simulink library "car_library"  (R2019b)
settings: Solver=VariableStepAuto  StartTime=0.0  StopTime=10.0  RelTol=1e-3
undefined symbols (not defined in the file): car, car_init
libraries: simulink x2, $bdroot x2
settings Model: Creator=ciba  LastModifiedBy=LongLongMagnumDong
settings DataIOCC: ReturnWorkspaceOutputs=off
settings DebuggingCC: ArithmeticOperatorsInVariantConditions=warning
settings SFSimCC: SimUseLocalCustomCode=off  CustomCodeUndefinedFunction=UseInterfaceOnly
settings RTWCC: RTWUseLocalCustomCode=off
settings CodeAppCC: StateflowObjectComments=on

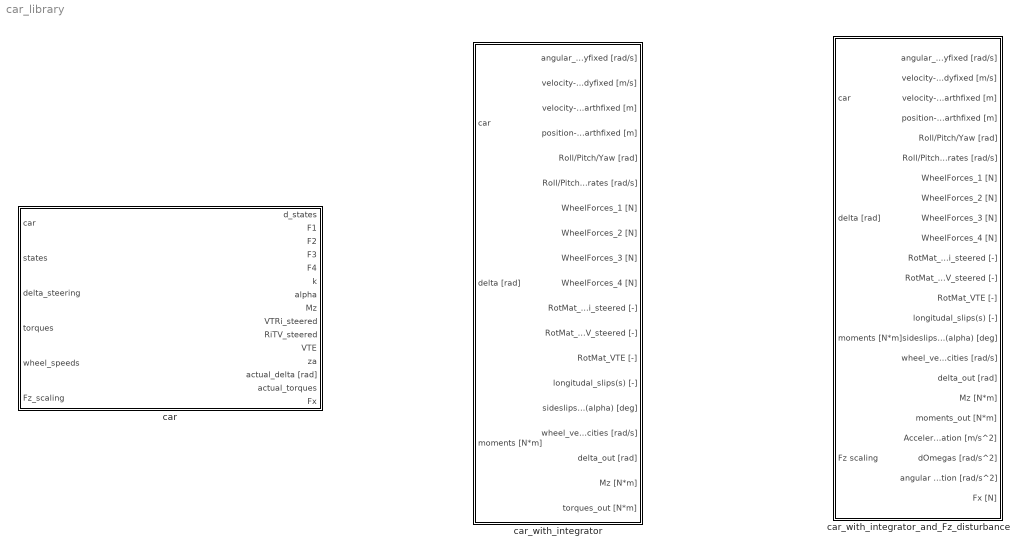
== system car_library ==
  car : Subsystem
  car_with_integrator : Subsystem
  car_with_integrator_and_Fz_disturbance : Subsystem

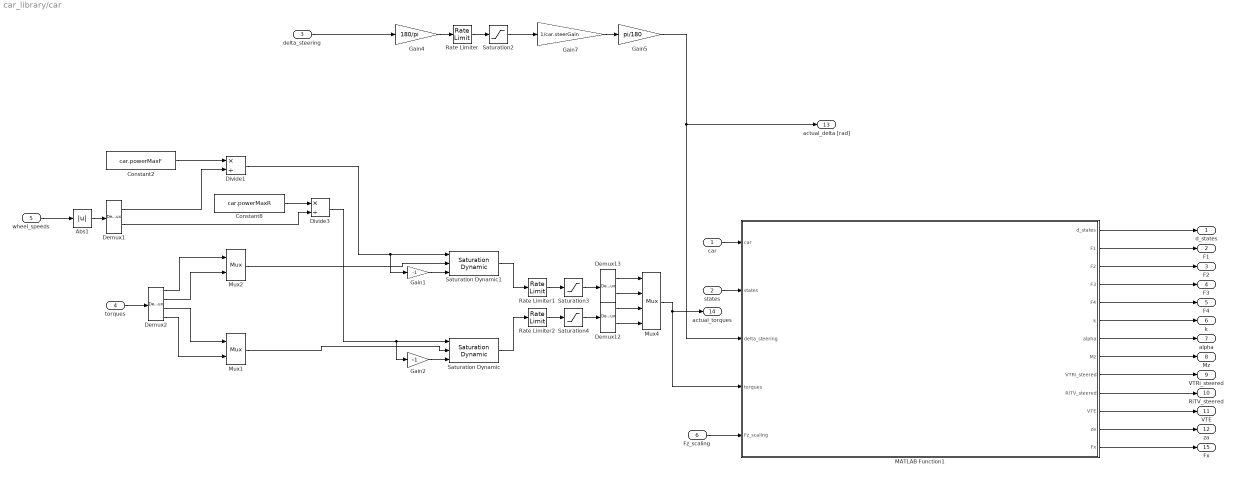
== system car_library/car ==
  car : Inport
  states : Inport  Port=2
  delta_steering : Inport  Port=3  PortDimensions=4
  torques : Inport  Port=4
  wheel_speeds : Inport  Port=5
  Fz_scaling : Inport  Port=6
  Abs1 : Abs
  Constant2 : Constant  Value=car.powerMaxF
  Constant8 : Constant  Value=car.powerMaxR
  Demux1 : Demux  Outputs=2
  Demux12 : Demux  Outputs=2
  Demux13 : Demux  Outputs=2
  Demux2 : Demux
  Divide1 : Product  Inputs=*/
  Divide3 : Product  Inputs=*/
  Gain1 : Gain  Gain=-1
  Gain2 : Gain  Gain=-1
  Gain4 : Gain  Gain=180/pi
  Gain5 : Gain  Gain=pi/180
  Gain7 : Gain  Gain=1/car.steerGain
  MATLAB Function1 : MATLAB Function  TreatAsAtomicUnit=on
  Mux1 : Mux  Inputs=2
  Mux2 : Mux  Inputs=2
  Mux4 : Mux
  Rate Limiter : RateLimiter  RisingSlewLimit=car.steerRate  FallingSlewLimit=-car.steerRate  SampleTimeMode=inherited
  Rate Limiter1 : RateLimiter  RisingSlewLimit=car.torqueRate  FallingSlewLimit=-car.torqueRate  SampleTimeMode=inherited
  Rate Limiter2 : RateLimiter  RisingSlewLimit=car.torqueRate  FallingSlewLimit=-car.torqueRate  SampleTimeMode=inherited
  Saturation Dynamic : simulink/Discontinuities/Saturation Dynamic  OutMin=[]  OutMax=[]  OutDataTypeStr=Inherit: Same as second input  OutDataType=fixdt(1, 16)  OutScaling=2^-10  DoSatur=off
  Saturation Dynamic1 : simulink/Discontinuities/Saturation Dynamic  OutMin=[]  OutMax=[]  OutDataTypeStr=Inherit: Same as second input  OutDataType=fixdt(1, 16)  OutScaling=2^-10  DoSatur=off
  Saturation2 : Saturate  UpperLimit=car.steerMaxDeg  LowerLimit=-car.steerMaxDeg
  Saturation3 : Saturate  UpperLimit=car.torqueMaxF  LowerLimit=-car.torqueMaxF
  Saturation4 : Saturate  UpperLimit=car.torqueMaxR  LowerLimit=-car.torqueMaxR
  d_states : Outport  VectorParamsAs1DForOutWhenUnconnected=off
  F1 : Outport  Port=2  VectorParamsAs1DForOutWhenUnconnected=off
  F2 : Outport  Port=3  VectorParamsAs1DForOutWhenUnconnected=off
  F3 : Outport  Port=4  VectorParamsAs1DForOutWhenUnconnected=off
  F4 : Outport  Port=5  VectorParamsAs1DForOutWhenUnconnected=off
  k : Outport  Port=6  VectorParamsAs1DForOutWhenUnconnected=off
  alpha : Outport  Port=7  VectorParamsAs1DForOutWhenUnconnected=off
  Mz : Outport  Port=8  VectorParamsAs1DForOutWhenUnconnected=off
  VTRi_steered : Outport  Port=9  VectorParamsAs1DForOutWhenUnconnected=off
  RiTV_steered : Outport  Port=10  VectorParamsAs1DForOutWhenUnconnected=off
  VTE : Outport  Port=11  VectorParamsAs1DForOutWhenUnconnected=off
  za : Outport  Port=12  VectorParamsAs1DForOutWhenUnconnected=off
  actual_delta [rad] : Outport  Port=13  VectorParamsAs1DForOutWhenUnconnected=off
  actual_torques : Outport  Port=14  VectorParamsAs1DForOutWhenUnconnected=off
  Fx : Outport  Port=15  VectorParamsAs1DForOutWhenUnconnected=off
  wires:
  Rate Limiter2/1 -> Saturation4/1
  Demux12/1 -> Mux4/3
  Saturation3/1 -> Demux13/1
  Demux1/2 -> Divide3/2
  Saturation4/1 -> Demux12/1
  Mux1/1 -> Saturation Dynamic/2
  Demux12/2 -> Mux4/4
  Demux2/1 -> Mux2/1
  Demux13/1 -> Mux4/1
  Saturation Dynamic/1 -> Rate Limiter2/1
  Rate Limiter1/1 -> Saturation3/1
  Demux13/2 -> Mux4/2
  Constant8/1 -> Divide3/1
  Abs1/1 -> Demux1/1
  Mux4/1 -> MATLAB Function1/4(torques), actual_torques/1
  car/1 -> MATLAB Function1/1(car)
  states/1 -> MATLAB Function1/2(states)
  MATLAB Function1/2(F1) -> F1/1
  MATLAB Function1/6(k) -> k/1
  MATLAB Function1/12(za) -> za/1
  MATLAB Function1/10(RiTV_steered) -> RiTV_steered/1
  MATLAB Function1/11(VTE) -> VTE/1
  MATLAB Function1/4(F3) -> F3/1
  torques/1 -> Demux2/1
  MATLAB Function1/1(d_states) -> d_states/1
  MATLAB Function1/3(F2) -> F2/1
  MATLAB Function1/9(VTRi_steered) -> VTRi_steered/1
  MATLAB Function1/8(Mz) -> Mz/1
  MATLAB Function1/5(F4) -> F4/1
  MATLAB Function1/7(alpha) -> alpha/1
  Demux2/4 -> Mux1/2
  Saturation Dynamic1/1 -> Rate Limiter1/1
  Mux2/1 -> Saturation Dynamic1/2
  Demux2/2 -> Mux2/2
  Constant2/1 -> Divide1/1
  Divide1/1 -> Gain1/1, Saturation Dynamic1/1
  wheel_speeds/1 -> Abs1/1
  Demux2/3 -> Mux1/1
  Gain4/1 -> Rate Limiter/1
  delta_steering/1 -> Gain4/1
  Saturation2/1 -> Gain7/1
  Rate Limiter/1 -> Saturation2/1
  Gain7/1 -> Gain5/1
  Gain1/1 -> Saturation Dynamic1/3
  Divide3/1 -> Gain2/1, Saturation Dynamic/1
  Gain2/1 -> Saturation Dynamic/3
  Demux1/1 -> Divide1/2
  Gain5/1 -> actual_delta [rad]/1, MATLAB Function1/3(delta_steering)
  Fz_scaling/1 -> MATLAB Function1/5(Fz_scaling)
  MATLAB Function1/13(Fx) -> Fx/1

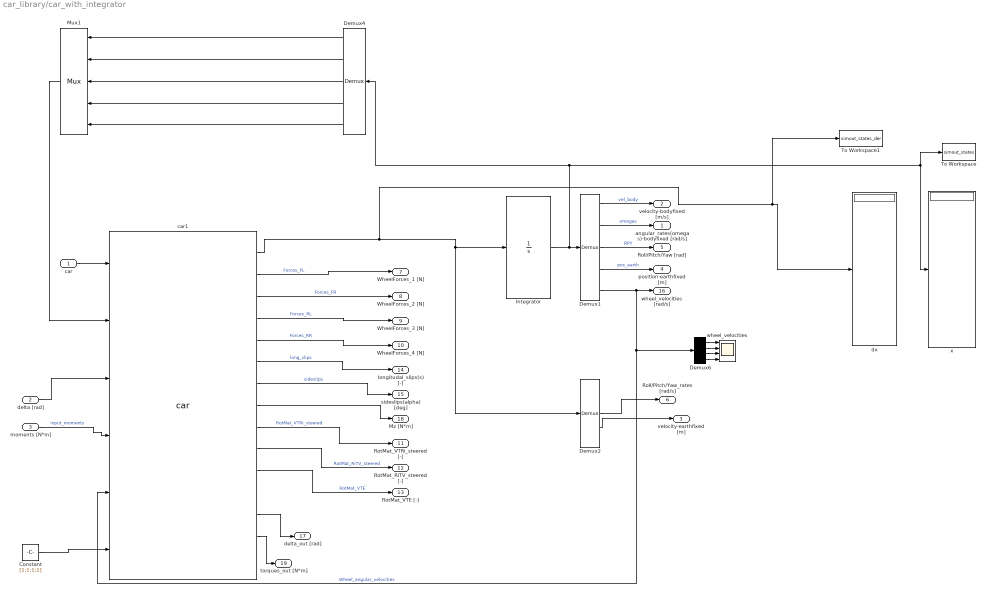
== system car_library/car_with_integrator ==
  car : Inport
  delta [rad] : Inport  Port=2  Unit=rad
  moments [N*m] : Inport  Port=3  Unit=N*m
  Constant : Constant  Value=[1;1;1;1]
  Demux1 : Demux  Outputs=[3,3,3,3,4]
  Demux2 : Demux  Outputs=[3,3,3,3,4]
  Demux4 : Demux  Outputs=[3,3,3,3,4]
  Demux6 : Demux
  Integrator : Integrator  InitialCondition=car_init(1:16)
  Mux1 : Mux  Inputs=5
  To Workspace : ToWorkspace  VariableName=simout_states  SampleTime=-1
  To Workspace1 : ToWorkspace  VariableName=simout_states_der  SampleTime=-1
  car1 : $bdroot/car  SystemSampleTime=-1  Latency=0  AutoFrameSizeCalculation=off
  dx : Display
  wheel_velocities : Scope  NumInputPorts=4
  x : Display
  angular_rates(omegas)-bodyfixed [rad/s] : Outport  PortDimensions=3  VectorParamsAs1DForOutWhenUnconnected=off
  velocity-bodyfixed [m/s] : Outport  Port=2  PortDimensions=3  VectorParamsAs1DForOutWhenUnconnected=off
  velocity-earthfixed [m] : Outport  Port=3  PortDimensions=3  VectorParamsAs1DForOutWhenUnconnected=off
  position-earthfixed [m] : Outport  Port=4  PortDimensions=3  VectorParamsAs1DForOutWhenUnconnected=off
  Roll/Pitch/Yaw [rad] : Outport  Port=5  PortDimensions=3  VectorParamsAs1DForOutWhenUnconnected=off
  Roll/Pitch/Yaw_rates [rad/s] : Outport  Port=6  PortDimensions=3  VectorParamsAs1DForOutWhenUnconnected=off
  WheelForces_1 [N] : Outport  Port=7  VectorParamsAs1DForOutWhenUnconnected=off
  WheelForces_2 [N] : Outport  Port=8  VectorParamsAs1DForOutWhenUnconnected=off
  WheelForces_3 [N] : Outport  Port=9  VectorParamsAs1DForOutWhenUnconnected=off
  WheelForces_4 [N] : Outport  Port=10  VectorParamsAs1DForOutWhenUnconnected=off
  RotMat_VTRi_steered [-] : Outport  Port=11  VectorParamsAs1DForOutWhenUnconnected=off
  RotMat_RiTV_steered [-] : Outport  Port=12  VectorParamsAs1DForOutWhenUnconnected=off
  RotMat_VTE [-] : Outport  Port=13  VectorParamsAs1DForOutWhenUnconnected=off
  longitudal_slips(s) [-] : Outport  Port=14  VectorParamsAs1DForOutWhenUnconnected=off
  sideslips(alpha) [deg] : Outport  Port=15  VectorParamsAs1DForOutWhenUnconnected=off
  wheel_velocities [rad/s] : Outport  Port=16  VectorParamsAs1DForOutWhenUnconnected=off
  delta_out [rad] : Outport  Port=17  VectorParamsAs1DForOutWhenUnconnected=off
  Mz [N*m] : Outport  Port=18  VectorParamsAs1DForOutWhenUnconnected=off
  torques_out [N*m] : Outport  Port=19  VectorParamsAs1DForOutWhenUnconnected=off
  wires:
  Demux1/5 -> car1/5, Demux6/1, wheel_velocities [rad/s]/1  "Wheel_angular_velocities"
  car1/5 -> WheelForces_4 [N]/1  "Forces_RR"
  car1/3 -> WheelForces_2 [N]/1  "Forces_FR"
  car1/2 -> WheelForces_1 [N]/1  "Forces_FL"
  car1/4 -> WheelForces_3 [N]/1  "Forces_RL"
  car1/11 -> RotMat_VTE [-]/1  "RotMat_VTE"
  delta [rad]/1 -> car1/3
  car1/7 -> sideslips(alpha) [deg]/1  "sideslips"
  car1/6 -> longitudal_slips(s) [-]/1  "long_slips"
  Demux1/3 -> Roll/Pitch/Yaw [rad]/1  "RPY"
  car1/9 -> RotMat_VTRi_steered [-]/1  "RotMat_VTRi_steered"
  Demux1/2 -> angular_rates(omegas)-bodyfixed [rad/s]/1  "omegas"
  Demux1/4 -> position-earthfixed [m]/1  "pos_earth"
  Demux1/1 -> velocity-bodyfixed [m/s]/1  "vel_body"
  moments [N*m]/1 -> car1/4  "input_moments"
  car1/10 -> RotMat_RiTV_steered [-]/1  "RotMat_RiTV_steered"
  Integrator/1 -> Demux4/1, x/1, To Workspace/1, Demux1/1
  car1/8 -> Mz [N*m]/1
  Demux2/4 -> velocity-earthfixed [m]/1
  Demux2/3 -> Roll/Pitch/Yaw_rates [rad/s]/1
  car1/13 -> delta_out [rad]/1
  car1/14 -> torques_out [N*m]/1
  Mux1/1 -> car1/2
  car1/1 -> Demux2/1, Integrator/1, To Workspace1/1, dx/1
  Demux4/1 -> Mux1/1
  Demux4/2 -> Mux1/2
  Demux4/3 -> Mux1/3
  Demux4/4 -> Mux1/4
  Demux4/5 -> Mux1/5
  Demux6/1 -> wheel_velocities/1
  Demux6/2 -> wheel_velocities/2
  Demux6/3 -> wheel_velocities/3
  Demux6/4 -> wheel_velocities/4
  car/1 -> car1/1
  Constant/1 -> car1/6

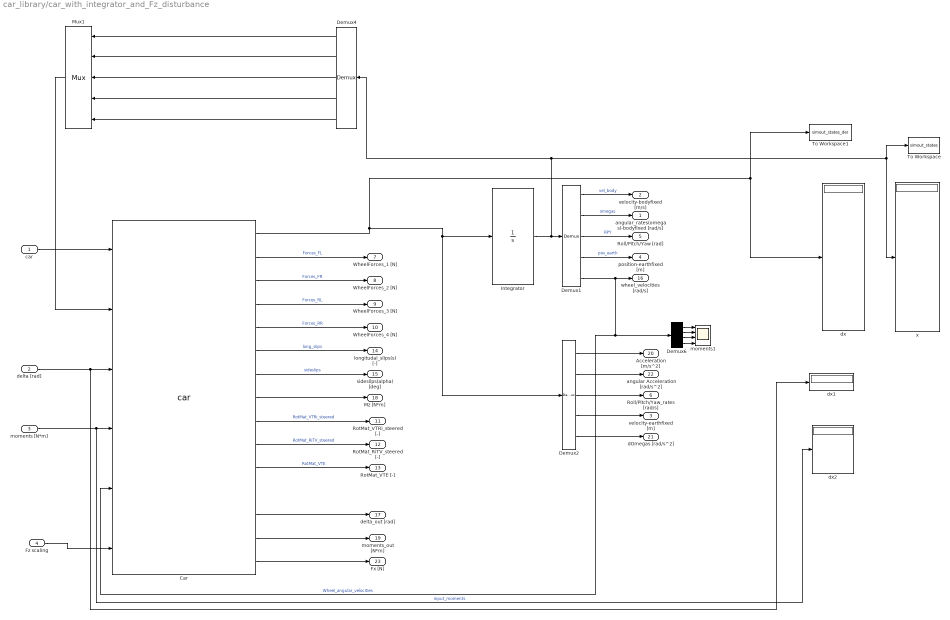
== system car_library/car_with_integrator_and_Fz_disturbance ==
  car : Inport
  delta [rad] : Inport  Port=2  Unit=rad
  moments [N*m] : Inport  Port=3  Unit=N*m
  Fz scaling : Inport  Port=4
  Car : $bdroot/car  SystemSampleTime=-1  Latency=0  AutoFrameSizeCalculation=off
  Demux1 : Demux  Outputs=[3,3,3,3,4]
  Demux2 : Demux  Outputs=[3,3,3,3,4]
  Demux4 : Demux  Outputs=[3,3,3,3,4]
  Demux6 : Demux
  Integrator : Integrator  InitialCondition=car_init(1:16)
  Mux1 : Mux  Inputs=5
  To Workspace : ToWorkspace  VariableName=simout_states  SampleTime=-1
  To Workspace1 : ToWorkspace  VariableName=simout_states_der  SampleTime=-1
  dx : Display
  dx1 : Display
  dx2 : Display
  moments1 : Scope  NumInputPorts=4
  x : Display
  angular_rates(omegas)-bodyfixed [rad/s] : Outport  PortDimensions=3  VectorParamsAs1DForOutWhenUnconnected=off
  velocity-bodyfixed [m/s] : Outport  Port=2  PortDimensions=3  VectorParamsAs1DForOutWhenUnconnected=off
  velocity-earthfixed [m] : Outport  Port=3  PortDimensions=3  VectorParamsAs1DForOutWhenUnconnected=off
  position-earthfixed [m] : Outport  Port=4  PortDimensions=3  VectorParamsAs1DForOutWhenUnconnected=off
  Roll/Pitch/Yaw [rad] : Outport  Port=5  PortDimensions=3  VectorParamsAs1DForOutWhenUnconnected=off
  Roll/Pitch/Yaw_rates [rad/s] : Outport  Port=6  PortDimensions=3  VectorParamsAs1DForOutWhenUnconnected=off
  WheelForces_1 [N] : Outport  Port=7  VectorParamsAs1DForOutWhenUnconnected=off
  WheelForces_2 [N] : Outport  Port=8  VectorParamsAs1DForOutWhenUnconnected=off
  WheelForces_3 [N] : Outport  Port=9  VectorParamsAs1DForOutWhenUnconnected=off
  WheelForces_4 [N] : Outport  Port=10  VectorParamsAs1DForOutWhenUnconnected=off
  RotMat_VTRi_steered [-] : Outport  Port=11  VectorParamsAs1DForOutWhenUnconnected=off
  RotMat_RiTV_steered [-] : Outport  Port=12  VectorParamsAs1DForOutWhenUnconnected=off
  RotMat_VTE [-] : Outport  Port=13  VectorParamsAs1DForOutWhenUnconnected=off
  longitudal_slips(s) [-] : Outport  Port=14  VectorParamsAs1DForOutWhenUnconnected=off
  sideslips(alpha) [deg] : Outport  Port=15  VectorParamsAs1DForOutWhenUnconnected=off
  wheel_velocities [rad/s] : Outport  Port=16  VectorParamsAs1DForOutWhenUnconnected=off
  delta_out [rad] : Outport  Port=17  VectorParamsAs1DForOutWhenUnconnected=off
  Mz [N*m] : Outport  Port=18  VectorParamsAs1DForOutWhenUnconnected=off
  moments_out [N*m] : Outport  Port=19  VectorParamsAs1DForOutWhenUnconnected=off
  Acceleration [m/s^2] : Outport  Port=20  PortDimensions=3  VectorParamsAs1DForOutWhenUnconnected=off
  dOmegas [rad/s^2] : Outport  Port=21  PortDimensions=4  VectorParamsAs1DForOutWhenUnconnected=off
  angular Acceleration [rad/s^2] : Outport  Port=22  PortDimensions=3  VectorParamsAs1DForOutWhenUnconnected=off
  Fx [N] : Outport  Port=23  VectorParamsAs1DForOutWhenUnconnected=off
  wires:
  car/1 -> Car/1
  Demux6/4 -> moments1/4
  Demux6/3 -> moments1/3
  Demux6/2 -> moments1/2
  Demux6/1 -> moments1/1
  Demux4/5 -> Mux1/5
  Demux4/4 -> Mux1/4
  Demux4/3 -> Mux1/3
  Demux4/2 -> Mux1/2
  Demux4/1 -> Mux1/1
  Car/1 -> dx/1, To Workspace1/1, Demux2/1, Integrator/1
  Mux1/1 -> Car/2
  Car/14 -> moments_out [N*m]/1
  Car/13 -> delta_out [rad]/1
  Demux2/3 -> Roll/Pitch/Yaw_rates [rad/s]/1
  Demux2/4 -> velocity-earthfixed [m]/1
  Car/8 -> Mz [N*m]/1
  Integrator/1 -> Demux1/1, To Workspace/1, x/1, Demux4/1
  Car/10 -> RotMat_RiTV_steered [-]/1  "RotMat_RiTV_steered"
  moments [N*m]/1 -> Car/4, dx2/1  "input_moments"
  Demux1/1 -> velocity-bodyfixed [m/s]/1  "vel_body"
  Demux1/4 -> position-earthfixed [m]/1  "pos_earth"
  Demux1/2 -> angular_rates(omegas)-bodyfixed [rad/s]/1  "omegas"
  Car/9 -> RotMat_VTRi_steered [-]/1  "RotMat_VTRi_steered"
  Demux1/3 -> Roll/Pitch/Yaw [rad]/1  "RPY"
  Car/6 -> longitudal_slips(s) [-]/1  "long_slips"
  Car/7 -> sideslips(alpha) [deg]/1  "sideslips"
  delta [rad]/1 -> Car/3, dx1/1
  Car/11 -> RotMat_VTE [-]/1  "RotMat_VTE"
  Car/4 -> WheelForces_3 [N]/1  "Forces_RL"
  Car/2 -> WheelForces_1 [N]/1  "Forces_FL"
  Car/3 -> WheelForces_2 [N]/1  "Forces_FR"
  Car/5 -> WheelForces_4 [N]/1  "Forces_RR"
  Demux1/5 -> wheel_velocities [rad/s]/1, Car/5, Demux6/1  "Wheel_angular_velocities"
  Fz scaling/1 -> Car/6
  Demux2/1 -> Acceleration [m/s^2]/1
  Demux2/5 -> dOmegas [rad/s^2]/1
  Demux2/2 -> angular Acceleration [rad/s^2]/1
  Car/15 -> Fx [N]/1

== matlab function car_library/car/MATLAB Function1 ==
  data: car input Bus: car_bus; d_states output size=16; states input size=16; delta_steering input size=4; F1 output size=3; F2 output size=3; F3 output size=3; F4 output size=3; k output size=4; alpha output size=4; Mz output size=4; VTRi_steered output size=[3,3]; RiTV_steered output size=[3,3]; VTE output size=[3,3]; za output size=4; torques input size=4; Fz_scaling input size=4; Fx output
function [ d_states,F1,F2,F3,F4,k,alpha,Mz,VTRi_steered,RiTV_steered,VTE,za, Fx ] ...
    = twintrack( car,states,delta_steering,torques, Fz_scaling )

[ d_states,F_R,k,alpha,Mz,VTRi_steered,RiTV_steered,VTE,za, ~, ~, ~, Fx ] ...
    = twintrack( car,states,delta_steering,torques, Fz_scaling);

F1 = F_R(:,1);
F2 = F_R(:,2);
F3 = F_R(:,3);
F4 = F_R(:,4);
